simulink model "Single_Phase_VSR_Simulation"  (R2022b)
settings: Solver=FixedStepDiscrete  StartTime=0.0  StopTime=0.6  FixedStep=1e-6  RelTol=1e-3
libraries: spsSeriesRLCBranchLib x10, spsCurrentMeasurementLib x4, spsMosfetLib x4, slpidlib x3, spsRMSLib x3, simulink x3, spsVoltageMeasurementLib x3, spsFourierLib x2, spsMeanLib x2, spsIdealSwitchLib x1, spspowerguiLib x1, spsControlledVoltageSourceLib x1
(part 2 of 2)

== matlab function Single_Phase_VSR_Simulation/MATLAB Function17 ==
  settings: updateMethod=DISCRETE
  data: U_in input; U_prime output; deltaU_prime output
function [U_prime, deltaU_prime] = SOGI_FLL_Process(U_in)
% SOGI-FLL for Simulink: 逐点更新，内置相位积分，维护状态记忆
% 输入：U_in   - 当前时刻输入电压（标量）
% 输出：U_prime      - α轴同相输出（标量）
%       deltaU_prime - β轴正交输出（标量）
%       omega0       - 当前角频率（rad/s，标量）
%       theta        - 积分得到的瞬时相位（rad，标量，θ=∫ωdt）

%% 固定参数
dt = 1e-5;               % 仿真步长，必须与Simulink求解器步长一致
K = 1.414;               % SOGI增益
K1 = 0.25;               % 直流消除器增益
gamma = 20;              % FLL增益（你已调至46，加快收敛）
omega0_init = 100*pi;    % 初始角频率（50Hz）
w_max = 2*pi*60;         % 频率上限（60Hz）
w_min = 2*pi*40;         % 频率下限（40Hz）

%% 状态变量持久化（Simulink中必须用persistent）
persistent x1_prev x2_prev x3_prev omega0_prev theta_prev first_run

if isempty(first_run)
    % 首次运行初始化
    x1_prev = 0;
    x2_prev = 0;
    x3_prev = 0;
    omega0_prev = omega0_init;
    theta_prev = 0;       % 相位积分初始值（θ₀=0，匹配输入无初相）
    first_run = false;
end

%% 1. 计算状态导数（逐点，无矩阵）
A11 = -K1 * omega0_prev; A12 = -K1 * omega0_prev; A13 = 0;
A21 = -K  * omega0_prev; A22 = -K  * omega0_prev; A23 = -omega0_prev^2;
A31 = 0;                  A32 = 1;                   A33 = 0;

B1 = K1 * omega0_prev;
B2 = K  * omega0_prev;
B3 = 0;

dx1dt = A11*x1_prev + A12*x2_prev + A13*x3_prev + B1*U_in;
dx2dt = A21*x1_prev + A22*x2_prev + A23*x3_prev + B2*U_in;
dx3dt = A31*x1_prev + A32*x2_prev + A33*x3_prev + B3*U_in;

%% 2. 前向欧拉更新状态
x1_curr = x1_prev + dt * dx1dt;
x2_curr = x2_prev + dt * dx2dt;
x3_curr = x3_prev + dt * dx3dt;

%% 3. FLL频率更新
deltaU = U_in - x1_curr - x2_curr;
deltaU_prime_k = omega0_prev * x3_curr;
epsilon_f = deltaU * deltaU_prime_k;
domega0dt = -gamma * epsilon_f;
omega0_curr = omega0_prev + dt * domega0dt;

% 频率限幅
omega0_curr = max(min(omega0_curr, w_max), w_min);

%% 4. 内置相位积分（梯形积分，精度更高）
% 梯形积分：theta = theta_prev + (当前ω + 前一时刻ω) * dt / 2
theta_curr = theta_prev + (omega0_curr + omega0_prev) * dt / 2;
% 相位归一化（限制在[-π, π]，避免数值溢出）
theta_curr = mod(theta_curr + pi, 2*pi) - pi;

%% 5. 输出
U_prime = x2_curr;
deltaU_prime = omega0_prev * x3_curr;  % 用前一时刻ω₀计算正交分量
omega0 = omega0_curr;
theta = theta_curr;  % 新增相位输出

%% 6. 更新状态，供下一时刻使用
x1_prev = x1_curr;
x2_prev = x2_curr;
x3_prev = x3_curr;
omega0_prev = omega0_curr;
theta_prev = theta_curr;  % 更新相位状态
end

== matlab function Single_Phase_VSR_Simulation/MATLAB Function18 ==
  data: u_alpha input; theta output; u_beta input; qerror output
function [theta, qerror] = SRF_PLL(u_alpha, u_beta)
% 同步旋转坐标系锁相环 SRF-PLL（严格匹配框图逻辑）
% 输入
%   u_alpha:  α轴输入信号（对应框图的v'，与电网电压同相）
%   u_beta:   β轴输入信号（对应框图的qv'，与电网电压正交90°）
% 输出
%   theta:    锁相得到的电网相位 [0, 2π)
%   qerror:   q轴相位误差（锁相锁定时趋近于0）
% 适配：仿真步长 Ts=1e-5（10kHz采样），基波频率50Hz

    %% ===================== 1. 固定参数配置 =====================
    Ts = 1e-5;               % 采样时间，必须与全局仿真步长完全一致
    f0 = 50;                  % 电网额定基波频率 (Hz)
    w0 = 2 * pi * f0;        % 额定角频率 (rad/s)
    
    % PI控制器参数（适配10kHz采样，可按需调整）
    kp_pll = 60;              % 比例系数：增大加快锁相响应，过大易振荡
    ki_pll = 5000;            % 积分系数：增大减小稳态相位误差，过大影响稳定性

    %% ===================== 2. 持久变量初始化（仅首次运行执行） =====================
    persistent theta_prev     % 上一拍的锁相相位
    persistent xi_pll         % PI控制器的积分项（抗饱和）
    
    if isempty(theta_prev)
        theta_prev = 0;       % 相位初始值清零
        xi_pll = 0;           % 积分项初始值清零
    end

    %% ===================== 3. αβ/dq 帕克变换（核心鉴相环节） =====================
    % 标准帕克变换矩阵，严格匹配框图逻辑
    % [u_d]   = [ cosθ   sinθ ] [u_alpha]
    % [u_q]     [ -sinθ  cosθ ] [u_beta ]
    cos_theta = cos(theta_prev);
    sin_theta = sin(theta_prev);
    
    u_d = u_alpha * cos_theta + u_beta * sin_theta;  % d轴分量（对应电压幅值）
    u_q = -u_alpha * sin_theta + u_beta * cos_theta; % q轴分量（相位误差）
    
    qerror = u_q; % 输出q轴相位误差，锁相锁定时qerror→0

    %% ===================== 4. PI环路控制器 =====================
    % 位置式PI控制器，带积分抗饱和
    xi_pll = xi_pll + ki_pll * Ts * qerror;  % 积分项更新
    delta_w = kp_pll * qerror + xi_pll;      % 频率偏差量
    w_pll = w0 + delta_w;                     % 锁相得到的实时角频率

    %% ===================== 5. 积分环节（1/s）生成相位 =====================
    % 前向欧拉离散化，对应框图的1/s积分环节
    theta = theta_prev + Ts * w_pll;
    
    % 相位归一化到 [0, 2π)，防止数值溢出
    theta = mod(theta, 2 * pi);

    %% ===================== 6. 更新状态变量（为下一拍迭代准备） =====================
    theta_prev = theta;

end

== matlab function Single_Phase_VSR_Simulation/级联谐波抑制3 ==
  data: u input; y output
function y = Cascade_Notch_Filter(u)
% 级联陷波滤波器：滤除3/5/7次固定频率谐波（150/250/350Hz）
% 输入u：待滤波的标量信号
% 输出y：滤波后的标量信号
% 适配：20kHz采样率（Ts=5e-5），和你的控制环完全对齐

    persistent x3_1 x3_2 x5_1 x5_2 x7_1 x7_2 first_run
    persistent b3_0 b3_1 b3_2 a3_1 a3_2
    persistent b5_0 b5_1 b5_2 a5_1 a5_2
    persistent b7_0 b7_1 b7_2 a7_1 a7_2

    %% ===================== 1. 初始化：仅首次运行 =====================
    if isempty(first_run)
        % --- 固定参数 ---
        Fs = 2e4;          % 采样频率 20kHz
        Ts = 1/Fs;            % 采样周期 5e-5s
        wc = 10;              % 截止角频率 25 rad/s
        
        % 目标谐波频率
        w3 = 2*pi*150;  % 3次谐波 150Hz
        w5 = 2*pi*250;  % 5次谐波 250Hz
        w7 = 2*pi*350;  % 7次谐波 350Hz

        % --- Tustin变换预计算系数 ---
        k = 2/Ts;
        k2 = k*k;

        % --- 3次滤波器系数 ---
        [b3_0, b3_1, b3_2, a3_1, a3_2] = calc_coeff(w3, wc, k, k2);
        % --- 5次滤波器系数 ---
        [b5_0, b5_1, b5_2, a5_1, a5_2] = calc_coeff(w5, wc, k, k2);
        % --- 7次滤波器系数 ---
        [b7_0, b7_1, b7_2, a7_1, a7_2] = calc_coeff(w7, wc, k, k2);

        % --- 显式初始化状态变量为标量 ---
        x3_1 = 0; x3_2 = 0;
        x5_1 = 0; x5_2 = 0;
        x7_1 = 0; x7_2 = 0;
        
        first_run = 1;
    end

    %% ===================== 2. 级联滤波计算（显式差分方程） =====================
    % --- 第1级：3次谐波滤波 ---
    y3 = b3_0*u + x3_1;
    x3_1_next = b3_1*u - a3_1*y3 + x3_2;
    x3_2_next = b3_2*u - a3_2*y3;
    
    % --- 第2级：5次谐波滤波 ---
    y5 = b5_0*y3 + x5_1;
    x5_1_next = b5_1*y3 - a5_1*y5 + x5_2;
    x5_2_next = b5_2*y3 - a5_2*y5;
    
    % --- 第3级：7次谐波滤波 ---
    y7 = b7_0*y5 + x7_1;
    x7_1_next = b7_1*y5 - a7_1*y7 + x7_2;
    x7_2_next = b7_2*y5 - a7_2*y7;
    
    % --- 更新状态变量 ---
    x3_1 = x3_1_next; x3_2 = x3_2_next;
    x5_1 = x5_1_next; x5_2 = x5_2_next;
    x7_1 = x7_1_next; x7_2 = x7_2_next;
    
    % --- 最终输出 ---
    y = y7;

end

%% ===================== 局部函数：预计算滤波器系数 =====================
function [b0, b1, b2, a1, a2] = calc_coeff(wn, wc, k, k2)
    % 连续域：G(s) = (s^2 + wn^2) / (s^2 + 2*wc*s + wn^2)
    % Tustin离散化：s = k*(z-1)/(z+1)
    
    % 连续域系数
    num_b0 = 1; num_b1 = 0; num_b2 = wn^2;
    den_a0 = 1; den_a1 = 2*wc; den_a2 = wn^2;
    
    % 离散化计算
    B0 = num_b0*k2 + num_b1*k + num_b2;
    B1 = 2*num_b2 - 2*num_b0*k2;
    B2 = num_b0*k2 - num_b1*k + num_b2;
    
    A0 = den_a0*k2 + den_a1*k + den_a2;
    A1 = 2*den_a2 - 2*den_a0*k2;
    A2 = den_a0*k2 - den_a1*k + den_a2;
    
    % 归一化（a0=1）
    b0 = B0 / A0;
    b1 = B1 / A0;
    b2 = B2 / A0;
    a1 = A1 / A0;
    a2 = A2 / A0;
end

== matlab function Single_Phase_VSR_Simulation/MATLAB Function ==
  data: i_error input; m output
function m  = QPR_Current_Loop(i_error)
% 单相LCL整流器 电流环 多谐振QPR控制器
% 【严格匹配论文公式】G = Kp + Σ(2Kr·wi·s)/(s²+2wi·s + wn²)
% 谐振项：基波50Hz + 3次150Hz +5次250Hz +7次350Hz
% 【参数规则】仅Kp全局共用，Kr/wi/w0 每项独立设置
% 采样率：20kHz | 双线性变换离散化

%% ===================== 独立历史变量 =====================
persistent e1_1 e1_2 m1_1 m1_2  % 基波 n=1
persistent e3_1 e3_2 m3_1 m3_2  % 3次  n=3
persistent e5_1 e5_2 m5_1 m5_2  % 5次  n=5
persistent e7_1 e7_2 m7_1 m7_2  % 7次  n=7

%% ===================== 全局共用参数（仅Kp） =====================
Ts    = 1/20000;   % 采样周期
Kp    = 0.6;       % 【唯一共用参数】比例增益

%% ===================== 各谐振项 独立参数（互不共用） =====================
% === 基波 50Hz (n=1) ===
Kr1 = 55;
wi1 = 15;
w01 = 100*pi;

% === 3次谐波 150Hz (n=3) ===
Kr3 = 55;
wi3 = 6;
w03 = 300*pi;

% === 5次谐波 250Hz (n=5) ===
Kr5 = 55;
wi5 = 6;
w05 = 500*pi;

% === 7次谐波 350Hz (n=7) ===
Kr7 = 55;
wi7 = 6;
w07 = 700*pi;

%% ===================== 初始化 =====================
if isempty(e1_1)
    e1_1=0;e1_2=0;m1_1=0;m1_2=0;
    e3_1=0;e3_2=0;m3_1=0;m3_2=0;
    e5_1=0;e5_2=0;m5_1=0;m5_2=0;
    e7_1=0;e7_2=0;m7_1=0;m7_2=0;
end

%% ===================== 1. 共用比例项 =====================
m_p = Kp * i_error;

%% ===================== 2. 基波谐振项计算 =====================
A1  = 2 * Kr1 * wi1;
B1  = 2 * wi1;
C1  = w01^2;
a0_1 = 4 + 2*B1*Ts + C1*Ts^2;
a1_1 = -8 + 2*C1*Ts^2;
a2_1 = 4 - 2*B1*Ts + C1*Ts^2;
b0_1 =  A1 * Ts;
b1_1 =  0;
b2_1 = -A1 * Ts;
m1 = (b0_1*i_error + b1_1*e1_1 + b2_1*e1_2 - a1_1*m1_1 - a2_1*m1_2) / a0_1;
% 更新
e1_2 = e1_1; e1_1 = i_error;
m1_2 = m1_1; m1_1 = m1;

%% ===================== 3. 3次谐波谐振项计算 =====================
A3  = 2 * Kr3 * wi3;
B3  = 2 * wi3;
C3  = w03^2;
a0_3 = 4 + 2*B3*Ts + C3*Ts^2;
a1_3 = -8 + 2*C3*Ts^2;
a2_3 = 4 - 2*B3*Ts + C3*Ts^2;
b0_3 =  A3 * Ts;
b1_3 =  0;
b2_3 = -A3 * Ts;
m3 = (b0_3*i_error + b1_3*e3_1 + b2_3*e3_2 - a1_3*m3_1 - a2_3*m3_2) / a0_3;
% 更新
e3_2 = e3_1; e3_1 = i_error;
m3_2 = m3_1; m3_1 = m3;

%% ===================== 4. 5次谐波谐振项计算 =====================
A5  = 2 * Kr5 * wi5;
B5  = 2 * wi5;
C5  = w05^2;
a0_5 = 4 + 2*B5*Ts + C5*Ts^2;
a1_5 = -8 + 2*C5*Ts^2;
a2_5 = 4 - 2*B5*Ts + C5*Ts^2;
b0_5 =  A5 * Ts;
b1_5 =  0;
b2_5 = -A5 * Ts;
m5 = (b0_5*i_error + b1_5*e5_1 + b2_5*e5_2 - a1_5*m5_1 - a2_5*m5_2) / a0_5;
% 更新
e5_2 = e5_1; e5_1 = i_error;
m5_2 = m5_1; m5_1 = m5;

%% ===================== 5. 7次谐波谐振项计算 =====================
A7  = 2 * Kr7 * wi7;
B7  = 2 * wi7;
C7  = w07^2;
a0_7 = 4 + 2*B7*Ts + C7*Ts^2;
a1_7 = -8 + 2*C7*Ts^2;
a2_7 = 4 - 2*B7*Ts + C7*Ts^2;
b0_7 =  A7 * Ts;
b1_7 =  0;
b2_7 = -A7 * Ts;
m7 = (b0_7*i_error + b1_7*e7_1 + b2_7*e7_2 - a1_7*m7_1 - a2_7*m7_2) / a0_7;
% 更新
e7_2 = e7_1; e7_1 = i_error;
m7_2 = m7_1; m7_1 = m7;

%% ===================== 总输出叠加 =====================
m = m_p + m1 + m3 + m5 + m7;

%% 可选限幅
% m = min(max(m, -1), 1);
end

== matlab function Single_Phase_VSR_Simulation/MATLAB Function20 ==
  data: i_error input; m output
function m  = QPR_Current_Loop(i_error)
% 单相LCL整流器 电流环 多谐振QPR控制器
% 【严格匹配论文公式】G = Kp + Σ(2Kr·wi·s)/(s²+2wi·s + wn²)
% 谐振项：基波50Hz + 3次150Hz +5次250Hz +7次350Hz
% 【参数规则】仅Kp全局共用，Kr/wi/w0 每项独立设置
% 采样率：20kHz | 双线性变换离散化

%% ===================== 独立历史变量 =====================
persistent e1_1 e1_2 m1_1 m1_2  % 基波 n=1
persistent e3_1 e3_2 m3_1 m3_2  % 3次  n=3
persistent e5_1 e5_2 m5_1 m5_2  % 5次  n=5
persistent e7_1 e7_2 m7_1 m7_2  % 7次  n=7

%% ===================== 全局共用参数（仅Kp） =====================
Ts    = 1/20000;   % 采样周期
Kp    = 0.6;       % 【唯一共用参数】比例增益

%% ===================== 各谐振项 独立参数（互不共用） =====================
% === 基波 50Hz (n=1) ===
Kr1 = 55;
wi1 = 15;
w01 = 100*pi;

% === 3次谐波 150Hz (n=3) ===
Kr3 = 55;
wi3 = 6;
w03 = 300*pi;

% === 5次谐波 250Hz (n=5) ===
Kr5 = 55;
wi5 = 6;
w05 = 500*pi;

% === 7次谐波 350Hz (n=7) ===
Kr7 = 55;
wi7 = 6;
w07 = 700*pi;

%% ===================== 初始化 =====================
if isempty(e1_1)
    e1_1=0;e1_2=0;m1_1=0;m1_2=0;
    e3_1=0;e3_2=0;m3_1=0;m3_2=0;
    e5_1=0;e5_2=0;m5_1=0;m5_2=0;
    e7_1=0;e7_2=0;m7_1=0;m7_2=0;
end

%% ===================== 1. 共用比例项 =====================
m_p = Kp * i_error;

%% ===================== 2. 基波谐振项计算 =====================
A1  = 2 * Kr1 * wi1;
B1  = 2 * wi1;
C1  = w01^2;
a0_1 = 4 + 2*B1*Ts + C1*Ts^2;
a1_1 = -8 + 2*C1*Ts^2;
a2_1 = 4 - 2*B1*Ts + C1*Ts^2;
b0_1 =  A1 * Ts;
b1_1 =  0;
b2_1 = -A1 * Ts;
m1 = (b0_1*i_error + b1_1*e1_1 + b2_1*e1_2 - a1_1*m1_1 - a2_1*m1_2) / a0_1;
% 更新
e1_2 = e1_1; e1_1 = i_error;
m1_2 = m1_1; m1_1 = m1;

%% ===================== 3. 3次谐波谐振项计算 =====================
A3  = 2 * Kr3 * wi3;
B3  = 2 * wi3;
C3  = w03^2;
a0_3 = 4 + 2*B3*Ts + C3*Ts^2;
a1_3 = -8 + 2*C3*Ts^2;
a2_3 = 4 - 2*B3*Ts + C3*Ts^2;
b0_3 =  A3 * Ts;
b1_3 =  0;
b2_3 = -A3 * Ts;
m3 = (b0_3*i_error + b1_3*e3_1 + b2_3*e3_2 - a1_3*m3_1 - a2_3*m3_2) / a0_3;
% 更新
e3_2 = e3_1; e3_1 = i_error;
m3_2 = m3_1; m3_1 = m3;

%% ===================== 4. 5次谐波谐振项计算 =====================
A5  = 2 * Kr5 * wi5;
B5  = 2 * wi5;
C5  = w05^2;
a0_5 = 4 + 2*B5*Ts + C5*Ts^2;
a1_5 = -8 + 2*C5*Ts^2;
a2_5 = 4 - 2*B5*Ts + C5*Ts^2;
b0_5 =  A5 * Ts;
b1_5 =  0;
b2_5 = -A5 * Ts;
m5 = (b0_5*i_error + b1_5*e5_1 + b2_5*e5_2 - a1_5*m5_1 - a2_5*m5_2) / a0_5;
% 更新
e5_2 = e5_1; e5_1 = i_error;
m5_2 = m5_1; m5_1 = m5;

%% ===================== 5. 7次谐波谐振项计算 =====================
A7  = 2 * Kr7 * wi7;
B7  = 2 * wi7;
C7  = w07^2;
a0_7 = 4 + 2*B7*Ts + C7*Ts^2;
a1_7 = -8 + 2*C7*Ts^2;
a2_7 = 4 - 2*B7*Ts + C7*Ts^2;
b0_7 =  A7 * Ts;
b1_7 =  0;
b2_7 = -A7 * Ts;
m7 = (b0_7*i_error + b1_7*e7_1 + b2_7*e7_2 - a1_7*m7_1 - a2_7*m7_2) / a0_7;
% 更新
e7_2 = e7_1; e7_1 = i_error;
m7_2 = m7_1; m7_1 = m7;

%% ===================== 总输出叠加 =====================
m = m_p + m1 + m3 + m5 + m7;

%% 可选限幅
% m = min(max(m, -1), 1);
end

== matlab function Single_Phase_VSR_Simulation/合闸后再传入信号1 ==
  data: t input; Uref output; Udc input; Udc_error output
function [Uref, Udc_error] = Udc_Control_Logic(t, Udc)
% 单相整流器 直流母线电压 合闸综合控制逻辑
% 功能：
%   1. 0.15s合闸前：Uref=0，不计算误差（Udc_error=0）
%   2. 0.15s后：Uref直接跳变到40V，开始计算误差 Udc_error = 40 - Udc
% 输入：
%   t: 仿真时间
%   Udc: 实际直流母线电压测量值
% 输出：
%   Uref: 直流母线电压给定值
%   Udc_error: 电压误差 = Uref - Udc（合闸后才有值）

persistent V_target t_start;
if isempty(V_target)
    V_target =40;      % 目标电压，直接给50V
    t_start = 0.15;     % 合闸时间
end

%% 核心逻辑：时间分段控制
if t < t_start
    % === 阶段1：合闸前 ===
    Uref = 0;           % 电压给定为0
    Udc_error = 0;      % 不计算误差，避免误动作
else
    % === 阶段2：合闸后 ===
    Uref = V_target;    % 直接跳变到40V恒定
    Udc_error = Uref - Udc; % 立刻开始计算误差，投入闭环
end

end

== matlab function Single_Phase_VSR_Simulation/模仿开关控制3 ==
  data: t input; mod_out output; mod_in input
function mod_out = gate_mod_signal(t, mod_in)
% 功能：0.25s前输出0，0.25s后输出原调制波mod_in
% 输入 t: 仿真时间 (Clock模块)
% 输入 mod_in: 原始调制波信号
% 输出 mod_out: 带使能的调制波信号

t_start =0.15; % 合闸时间

if t < t_start
    mod_out = 0;          % 合闸前强制输出0
else
    mod_out = mod_in;      % 合闸后输出原调制波
end
end

== matlab function Single_Phase_VSR_Simulation/级联谐波抑制4 ==
  data: u input; y output
function y = Cascade_Notch_Filter(u)
% 级联陷波滤波器：滤除3/5/7次固定频率谐波（150/250/350Hz）
% 输入u：待滤波的标量信号
% 输出y：滤波后的标量信号
% 适配：20kHz采样率（Ts=5e-5），和你的控制环完全对齐

    persistent x3_1 x3_2 x5_1 x5_2 x7_1 x7_2 first_run
    persistent b3_0 b3_1 b3_2 a3_1 a3_2
    persistent b5_0 b5_1 b5_2 a5_1 a5_2
    persistent b7_0 b7_1 b7_2 a7_1 a7_2

    %% ===================== 1. 初始化：仅首次运行 =====================
    if isempty(first_run)
        % --- 固定参数 ---
        Fs = 1e5;          % 采样频率 100kHz
        Ts = 1/Fs;            % 采样周期 5e-5s
        wc = 10;              % 截止角频率 25 rad/s
        
        % 目标谐波频率
        w3 = 2*pi*150;  % 3次谐波 150Hz
        w5 = 2*pi*250;  % 5次谐波 250Hz
        w7 = 2*pi*350;  % 7次谐波 350Hz

        % --- Tustin变换预计算系数 ---
        k = 2/Ts;
        k2 = k*k;

        % --- 3次滤波器系数 ---
        [b3_0, b3_1, b3_2, a3_1, a3_2] = calc_coeff(w3, wc, k, k2);
        % --- 5次滤波器系数 ---
        [b5_0, b5_1, b5_2, a5_1, a5_2] = calc_coeff(w5, wc, k, k2);
        % --- 7次滤波器系数 ---
        [b7_0, b7_1, b7_2, a7_1, a7_2] = calc_coeff(w7, wc, k, k2);

        % --- 显式初始化状态变量为标量 ---
        x3_1 = 0; x3_2 = 0;
        x5_1 = 0; x5_2 = 0;
        x7_1 = 0; x7_2 = 0;
        
        first_run = 1;
    end

    %% ===================== 2. 级联滤波计算（显式差分方程） =====================
    % --- 第1级：3次谐波滤波 ---
    y3 = b3_0*u + x3_1;
    x3_1_next = b3_1*u - a3_1*y3 + x3_2;
    x3_2_next = b3_2*u - a3_2*y3;
    
    % --- 第2级：5次谐波滤波 ---
    y5 = b5_0*y3 + x5_1;
    x5_1_next = b5_1*y3 - a5_1*y5 + x5_2;
    x5_2_next = b5_2*y3 - a5_2*y5;
    
    % --- 第3级：7次谐波滤波 ---
    y7 = b7_0*y5 + x7_1;
    x7_1_next = b7_1*y5 - a7_1*y7 + x7_2;
    x7_2_next = b7_2*y5 - a7_2*y7;
    
    % --- 更新状态变量 ---
    x3_1 = x3_1_next; x3_2 = x3_2_next;
    x5_1 = x5_1_next; x5_2 = x5_2_next;
    x7_1 = x7_1_next; x7_2 = x7_2_next;
    
    % --- 最终输出 ---
    y = y7;

end

%% ===================== 局部函数：预计算滤波器系数 =====================
function [b0, b1, b2, a1, a2] = calc_coeff(wn, wc, k, k2)
    % 连续域：G(s) = (s^2 + wn^2) / (s^2 + 2*wc*s + wn^2)
    % Tustin离散化：s = k*(z-1)/(z+1)
    
    % 连续域系数
    num_b0 = 1; num_b1 = 0; num_b2 = wn^2;
    den_a0 = 1; den_a1 = 2*wc; den_a2 = wn^2;
    
    % 离散化计算
    B0 = num_b0*k2 + num_b1*k + num_b2;
    B1 = 2*num_b2 - 2*num_b0*k2;
    B2 = num_b0*k2 - num_b1*k + num_b2;
    
    A0 = den_a0*k2 + den_a1*k + den_a2;
    A1 = 2*den_a2 - 2*den_a0*k2;
    A2 = den_a0*k2 - den_a1*k + den_a2;
    
    % 归一化（a0=1）
    b0 = B0 / A0;
    b1 = B1 / A0;
    b2 = B2 / A0;
    a1 = A1 / A0;
    a2 = A2 / A0;
end

== matlab function Single_Phase_VSR_Simulation/合闸再给目标值 ==
  data: t input; V_amp output
function V_amp = voltage_amp_step(t)
% 功能：0.15s合闸，直接阶跃到40V
% 时间轴：
%   t < 0.15s：合闸前，输出0
%   t ≥ 0.15s：合闸后，直接输出40V

persistent V_target t_start;
if isempty(V_target)
    V_target = 40;      % 目标电压
    t_start =0.15;     % 合闸时间
end

% 核心逻辑
if t < t_start
    V_amp = 0;  % 合闸前：输出0
else
    V_amp = V_target; % 0.15s后：直接输出40V
end

end

== matlab function Single_Phase_VSR_Simulation/MATLAB Function2 ==
  data: IGm_total input; Igm_clean output
function Igm_clean = Notch_100Hz_IGm(IGm_total)
% 100Hz陷波滤波器，放在IGm求和后，滤除二次纹波
% 陷波频率100Hz，带宽6Hz，采样率20kHz
% 输入：IGm_total = IGm1 + IGm2
% 输出：Igm_clean = 滤除100Hz纹波后的纯直流信号

%% 历史变量
persistent x_prev1 x_prev2 y_prev1 y_prev2;

%% 固定参数
Ts = 1/20000;
f0 = 100;          % 陷波频率100Hz
bw = 6;            % 陷波带宽6Hz
w0 = 2*pi*f0;
wb = 2*pi*bw;

%% 双线性变换离散化系数
k = 2/Ts;
a0 = k^2 + wb*k + w0^2;
a1 = 2*(w0^2 - k^2);
a2 = k^2 - wb*k + w0^2;
b0 = k^2 + w0^2;
b1 = 2*(w0^2 - k^2);
b2 = k^2 + w0^2;

%% 归一化
b0 = b0/a0;
b1 = b1/a0;
b2 = b2/a0;
a1 = a1/a0;
a2 = a2/a0;

%% 初始化
if isempty(x_prev1)
    x_prev1 = 0; x_prev2 = 0;
    y_prev1 = 0; y_prev2 = 0;
end

%% 差分方程
Igm_clean = b0*IGm_total + b1*x_prev1 + b2*x_prev2 - a1*y_prev1 - a2*y_prev2;

%% 更新历史变量
x_prev2 = x_prev1;
x_prev1 = IGm_total;
y_prev2 = y_prev1;
y_prev1 = Igm_clean;

end

== matlab function Single_Phase_VSR_Simulation/MATLAB Function10 ==
  data: alpha input; d output; beta input; theta input; q output
function [d, q] = Park_Transform(alpha, beta, theta)
% Park变换模块（直接输入SOGI-FLL的theta，无内部积分）
% 输入：
%   alpha - α轴分量（SOGI-FLL的U_prime）
%   beta  - β轴分量（SOGI-FLL的deltaU_prime）
%   theta - 瞬时相位（SOGI-FLL直接输出的theta）
% 输出：
%   d         - d轴（直轴）分量
%   q         - q轴（交轴）分量
%   cos_theta - 相位θ的余弦值（新增输出）
%   sin_theta - 相位θ的正弦值（新增输出）

%% 核心计算
cos_theta = cos(theta);  % 相位θ的余弦值
sin_theta = sin(theta);  % 相位θ的正弦值


% 修正后的 Park 变换公式（d轴对齐同相分量 beta）
d =  alpha * cos_theta + beta * sin_theta;
q = -alpha * sin_theta + beta * cos_theta;
end

== matlab function Single_Phase_VSR_Simulation/MATLAB Function4 ==
  data: alpha input; d output; beta input; theta input; q output
function [d, q] = Park_Transform(alpha, beta, theta)
% Park变换模块（直接输入SOGI-FLL的theta，无内部积分）
% 输入：
%   alpha - α轴分量（SOGI-FLL的U_prime）
%   beta  - β轴分量（SOGI-FLL的deltaU_prime）
%   theta - 瞬时相位（SOGI-FLL直接输出的theta）
% 输出：
%   d         - d轴（直轴）分量
%   q         - q轴（交轴）分量
%   cos_theta - 相位θ的余弦值（新增输出）
%   sin_theta - 相位θ的正弦值（新增输出）

%% 核心计算
cos_theta = cos(theta);  % 相位θ的余弦值
sin_theta = sin(theta);  % 相位θ的正弦值


% 修正后的 Park 变换公式（d轴对齐同相分量 beta）
d =  alpha * cos_theta + beta * sin_theta;
q = -alpha * sin_theta + beta * cos_theta;
end

== matlab function Single_Phase_VSR_Simulation/MATLAB Function6 ==
  settings: updateMethod=DISCRETE
  data: U_in input; U_prime output; deltaU_prime output
function [U_prime, deltaU_prime] = SOGI_FLL_Process(U_in)
% SOGI-FLL for Simulink: 逐点更新，内置相位积分，维护状态记忆
% 输入：U_in   - 当前时刻输入电压（标量）
% 输出：U_prime      - α轴同相输出（标量）
%       deltaU_prime - β轴正交输出（标量）
%       omega0       - 当前角频率（rad/s，标量）
%       theta        - 积分得到的瞬时相位（rad，标量，θ=∫ωdt）

%% 固定参数
dt = 1e-5;               % 仿真步长，必须与Simulink求解器步长一致
K = 1.414;               % SOGI增益
K1 = 0.25;               % 直流消除器增益
gamma = 20;              % FLL增益（你已调至46，加快收敛）
omega0_init = 100*pi;    % 初始角频率（50Hz）
w_max = 2*pi*60;         % 频率上限（60Hz）
w_min = 2*pi*40;         % 频率下限（40Hz）

%% 状态变量持久化（Simulink中必须用persistent）
persistent x1_prev x2_prev x3_prev omega0_prev theta_prev first_run

if isempty(first_run)
    % 首次运行初始化
    x1_prev = 0;
    x2_prev = 0;
    x3_prev = 0;
    omega0_prev = omega0_init;
    theta_prev = 0;       % 相位积分初始值（θ₀=0，匹配输入无初相）
    first_run = false;
end

%% 1. 计算状态导数（逐点，无矩阵）
A11 = -K1 * omega0_prev; A12 = -K1 * omega0_prev; A13 = 0;
A21 = -K  * omega0_prev; A22 = -K  * omega0_prev; A23 = -omega0_prev^2;
A31 = 0;                  A32 = 1;                   A33 = 0;

B1 = K1 * omega0_prev;
B2 = K  * omega0_prev;
B3 = 0;

dx1dt = A11*x1_prev + A12*x2_prev + A13*x3_prev + B1*U_in;
dx2dt = A21*x1_prev + A22*x2_prev + A23*x3_prev + B2*U_in;
dx3dt = A31*x1_prev + A32*x2_prev + A33*x3_prev + B3*U_in;

%% 2. 前向欧拉更新状态
x1_curr = x1_prev + dt * dx1dt;
x2_curr = x2_prev + dt * dx2dt;
x3_curr = x3_prev + dt * dx3dt;

%% 3. FLL频率更新
deltaU = U_in - x1_curr - x2_curr;
deltaU_prime_k = omega0_prev * x3_curr;
epsilon_f = deltaU * deltaU_prime_k;
domega0dt = -gamma * epsilon_f;
omega0_curr = omega0_prev + dt * domega0dt;

% 频率限幅
omega0_curr = max(min(omega0_curr, w_max), w_min);

%% 4. 内置相位积分（梯形积分，精度更高）
% 梯形积分：theta = theta_prev + (当前ω + 前一时刻ω) * dt / 2
theta_curr = theta_prev + (omega0_curr + omega0_prev) * dt / 2;
% 相位归一化（限制在[-π, π]，避免数值溢出）
theta_curr = mod(theta_curr + pi, 2*pi) - pi;

%% 5. 输出
U_prime = x2_curr;
deltaU_prime = omega0_prev * x3_curr;  % 用前一时刻ω₀计算正交分量
omega0 = omega0_curr;
theta = theta_curr;  % 新增相位输出

%% 6. 更新状态，供下一时刻使用
x1_prev = x1_curr;
x2_prev = x2_curr;
x3_prev = x3_curr;
omega0_prev = omega0_curr;
theta_prev = theta_curr;  % 更新相位状态
end

== matlab function Single_Phase_VSR_Simulation/MATLAB Function7 ==
  data: u_alpha input; theta output; u_beta input; qerror output
function [theta, qerror] = SRF_PLL(u_alpha, u_beta)
% 同步旋转坐标系锁相环 SRF-PLL（严格匹配框图逻辑）
% 输入
%   u_alpha:  α轴输入信号（对应框图的v'，与电网电压同相）
%   u_beta:   β轴输入信号（对应框图的qv'，与电网电压正交90°）
% 输出
%   theta:    锁相得到的电网相位 [0, 2π)
%   qerror:   q轴相位误差（锁相锁定时趋近于0）
% 适配：仿真步长 Ts=1e-5（10kHz采样），基波频率50Hz

    %% ===================== 1. 固定参数配置 =====================
    Ts = 1e-5;               % 采样时间，必须与全局仿真步长完全一致
    f0 = 50;                  % 电网额定基波频率 (Hz)
    w0 = 2 * pi * f0;        % 额定角频率 (rad/s)
    
    % PI控制器参数（适配10kHz采样，可按需调整）
    kp_pll = 60;              % 比例系数：增大加快锁相响应，过大易振荡
    ki_pll = 5000;            % 积分系数：增大减小稳态相位误差，过大影响稳定性

    %% ===================== 2. 持久变量初始化（仅首次运行执行） =====================
    persistent theta_prev     % 上一拍的锁相相位
    persistent xi_pll         % PI控制器的积分项（抗饱和）
    
    if isempty(theta_prev)
        theta_prev = 0;       % 相位初始值清零
        xi_pll = 0;           % 积分项初始值清零
    end

    %% ===================== 3. αβ/dq 帕克变换（核心鉴相环节） =====================
    % 标准帕克变换矩阵，严格匹配框图逻辑
    % [u_d]   = [ cosθ   sinθ ] [u_alpha]
    % [u_q]     [ -sinθ  cosθ ] [u_beta ]
    cos_theta = cos(theta_prev);
    sin_theta = sin(theta_prev);
    
    u_d = u_alpha * cos_theta + u_beta * sin_theta;  % d轴分量（对应电压幅值）
    u_q = -u_alpha * sin_theta + u_beta * cos_theta; % q轴分量（相位误差）
    
    qerror = u_q; % 输出q轴相位误差，锁相锁定时qerror→0

    %% ===================== 4. PI环路控制器 =====================
    % 位置式PI控制器，带积分抗饱和
    xi_pll = xi_pll + ki_pll * Ts * qerror;  % 积分项更新
    delta_w = kp_pll * qerror + xi_pll;      % 频率偏差量
    w_pll = w0 + delta_w;                     % 锁相得到的实时角频率

    %% ===================== 5. 积分环节（1/s）生成相位 =====================
    % 前向欧拉离散化，对应框图的1/s积分环节
    theta = theta_prev + Ts * w_pll;
    
    % 相位归一化到 [0, 2π)，防止数值溢出
    theta = mod(theta, 2 * pi);

    %% ===================== 6. 更新状态变量（为下一拍迭代准备） =====================
    theta_prev = theta;

end

== matlab function Single_Phase_VSR_Simulation/合闸再给目标值1 ==
  data: t input; V_amp output
function V_amp = voltage_amp_step(t)
% 功能：0.15s合闸，直接阶跃到40V
% 时间轴：
%   t < 0.15s：合闸前，输出0
%   t ≥ 0.15s：合闸后，直接输出40V

persistent V_target t_start;
if isempty(V_target)
    V_target = 40;      % 目标电压
    t_start =0.15;     % 合闸时间
end

% 核心逻辑
if t < t_start
    V_amp = 0;  % 合闸前：输出0
else
    V_amp = V_target; % 0.15s后：直接输出40V
end

end

== matlab function Single_Phase_VSR_Simulation/MATLAB Function5 ==
  data: alpha input; d output; beta input; theta input; q output
function [d, q] = Park_Transform(alpha, beta, theta)
% Park变换模块（直接输入SOGI-FLL的theta，无内部积分）
% 输入：
%   alpha - α轴分量（SOGI-FLL的U_prime）
%   beta  - β轴分量（SOGI-FLL的deltaU_prime）
%   theta - 瞬时相位（SOGI-FLL直接输出的theta）
% 输出：
%   d         - d轴（直轴）分量
%   q         - q轴（交轴）分量
%   cos_theta - 相位θ的余弦值（新增输出）
%   sin_theta - 相位θ的正弦值（新增输出）

%% 核心计算
cos_theta = cos(theta);  % 相位θ的余弦值
sin_theta = sin(theta);  % 相位θ的正弦值


% 修正后的 Park 变换公式（d轴对齐同相分量 beta）
d =  alpha * cos_theta + beta * sin_theta;
q = -alpha * sin_theta + beta * cos_theta;
end

== matlab function Single_Phase_VSR_Simulation/MATLAB Function8 ==
  settings: updateMethod=DISCRETE
  data: U_in input; U_prime output; deltaU_prime output
function [U_prime, deltaU_prime] = SOGI_FLL_Process(U_in)
% SOGI-FLL for Simulink: 逐点更新，内置相位积分，维护状态记忆
% 输入：U_in   - 当前时刻输入电压（标量）
% 输出：U_prime      - α轴同相输出（标量）
%       deltaU_prime - β轴正交输出（标量）
%       omega0       - 当前角频率（rad/s，标量）
%       theta        - 积分得到的瞬时相位（rad，标量，θ=∫ωdt）

%% 固定参数
dt = 1e-5;               % 仿真步长，必须与Simulink求解器步长一致
K = 1.414;               % SOGI增益
K1 = 0.25;               % 直流消除器增益
gamma = 20;              % FLL增益（你已调至46，加快收敛）
omega0_init = 100*pi;    % 初始角频率（50Hz）
w_max = 2*pi*60;         % 频率上限（60Hz）
w_min = 2*pi*40;         % 频率下限（40Hz）

%% 状态变量持久化（Simulink中必须用persistent）
persistent x1_prev x2_prev x3_prev omega0_prev theta_prev first_run

if isempty(first_run)
    % 首次运行初始化
    x1_prev = 0;
    x2_prev = 0;
    x3_prev = 0;
    omega0_prev = omega0_init;
    theta_prev = 0;       % 相位积分初始值（θ₀=0，匹配输入无初相）
    first_run = false;
end

%% 1. 计算状态导数（逐点，无矩阵）
A11 = -K1 * omega0_prev; A12 = -K1 * omega0_prev; A13 = 0;
A21 = -K  * omega0_prev; A22 = -K  * omega0_prev; A23 = -omega0_prev^2;
A31 = 0;                  A32 = 1;                   A33 = 0;

B1 = K1 * omega0_prev;
B2 = K  * omega0_prev;
B3 = 0;

dx1dt = A11*x1_prev + A12*x2_prev + A13*x3_prev + B1*U_in;
dx2dt = A21*x1_prev + A22*x2_prev + A23*x3_prev + B2*U_in;
dx3dt = A31*x1_prev + A32*x2_prev + A33*x3_prev + B3*U_in;

%% 2. 前向欧拉更新状态
x1_curr = x1_prev + dt * dx1dt;
x2_curr = x2_prev + dt * dx2dt;
x3_curr = x3_prev + dt * dx3dt;

%% 3. FLL频率更新
deltaU = U_in - x1_curr - x2_curr;
deltaU_prime_k = omega0_prev * x3_curr;
epsilon_f = deltaU * deltaU_prime_k;
domega0dt = -gamma * epsilon_f;
omega0_curr = omega0_prev + dt * domega0dt;

% 频率限幅
omega0_curr = max(min(omega0_curr, w_max), w_min);

%% 4. 内置相位积分（梯形积分，精度更高）
% 梯形积分：theta = theta_prev + (当前ω + 前一时刻ω) * dt / 2
theta_curr = theta_prev + (omega0_curr + omega0_prev) * dt / 2;
% 相位归一化（限制在[-π, π]，避免数值溢出）
theta_curr = mod(theta_curr + pi, 2*pi) - pi;

%% 5. 输出
U_prime = x2_curr;
deltaU_prime = omega0_prev * x3_curr;  % 用前一时刻ω₀计算正交分量
omega0 = omega0_curr;
theta = theta_curr;  % 新增相位输出

%% 6. 更新状态，供下一时刻使用
x1_prev = x1_curr;
x2_prev = x2_curr;
x3_prev = x3_curr;
omega0_prev = omega0_curr;
theta_prev = theta_curr;  % 更新相位状态
end
